simulink model "prop2"  (R2015a)
settings: Solver=ode45  StartTime=0.0  StopTime=10.0  RelTol=1e-3
libraries: simulink x3, sldvlib x1
settings Model: Creator=teme  LastModifiedBy=teme

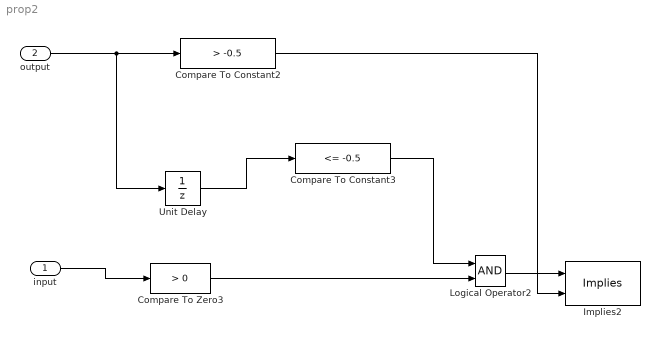
== system prop2 ==
  input : Inport
  output : Inport  Port=2
  Compare To Constant2 : simulink/Logic and Bit Operations/Compare To Constant  relop=>  const=-0.5  OutDataTypeStr=boolean
  Compare To Constant3 : simulink/Logic and Bit Operations/Compare To Constant  relop=<=  const=-0.5  OutDataTypeStr=boolean
  Compare To Zero3 : simulink/Logic and Bit Operations/Compare To Zero  relop=>  OutDataTypeStr=boolean
  Implies2 : sldvlib/Verification Utilities/Implies
  Logical Operator2 : Logic  AllPortsSameDT=off  OutDataTypeStr=boolean
  Unit Delay : UnitDelay  SampleTime=-1
  wires:
  output/1 -> Unit Delay/1, Compare To Constant2/1
  Unit Delay/1 -> Compare To Constant3/1
  input/1 -> Compare To Zero3/1
  Compare To Constant3/1 -> Logical Operator2/1
  Compare To Zero3/1 -> Logical Operator2/2
  Logical Operator2/1 -> Implies2/1
  Compare To Constant2/1 -> Implies2/2
